simulink model "radia_ltspice_pid_optuna"  (R2026a)
settings: Solver=FixedStepDiscrete  StopTime=0.80000000000000004  FixedStep=0.1
settings Model: Creator=Administrator  LastModifiedBy=Administrator

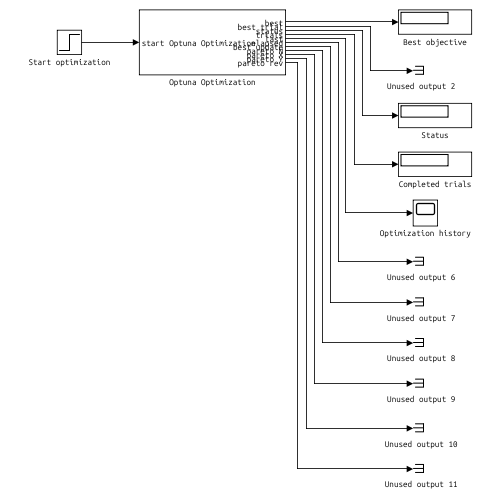
[thumbnail: Simulink's stored preview of the top-level diagram]
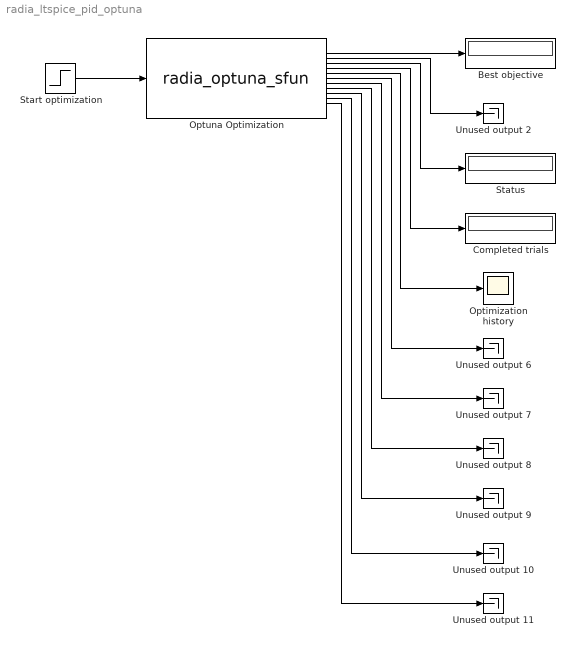
== system radia_ltspice_pid_optuna ==
  Best objective : Display
  Completed trials : Display
  Optimization history : Scope
  Optuna Optimization : M-S-Function  FunctionName=radia_optuna_sfun  Parameters=objective_fcn,num_trials,directions,storage_path,sample_time_s,strcmp(live_visualization,'on'),sampler_name  mask{objective_fcn='radia.simulink.ltspicePIDObjective', num_trials=8, directions="minimize", storage_path='', sample_time_s=0.10000000000000001, live_visualization=off, sampler_name=cmaes}
      mask prompts: objective_fcn "Objective function"; num_trials "Number of trials"; directions "Objective directions"; storage_path "Study MAT file"; sample_time_s "Trial sample time (s)"; live_visualization "External MATLAB monitor"; sampler_name "Sampler"
      mask help: Incremental MATLAB Optuna study. One trial executes per sample; connect the live outputs to an Optuna Monitor.
      mask TypeOptions sampler_name: auto | random | tpe | cmaes | motpe | nsgaii
      mask Display: disp('Optuna Optimization');port_label('input',1,'start');port_label('output',1,'best');port_label('output',2,'best trial');port_label('output',3,'status');port_label('output',4,'trials');port_label('output',5,'last');port_label('output',6,'elapsed');port_label('output',7,'best update');port_label('output',8,'pareto N');port_label('output',9,'pareto X');port_label('output',10,'pareto Y');port_label('output',11,'pareto rev');
  Start optimization : Step  Time=0  SampleTime=0.1
  Status : Display
  Unused output {2,6..11} (7 alike) : Terminator
  wires:
  Start optimization/1 -> Optuna Optimization/1
  Optuna Optimization/1 -> Best objective/1
  Optuna Optimization/2 -> Unused output 2/1
  Optuna Optimization/4 -> Completed trials/1
  Optuna Optimization/3 -> Status/1
  Optuna Optimization/10 -> Unused output 10/1
  Optuna Optimization/5 -> Optimization history/1
  Optuna Optimization/7 -> Unused output 7/1
  Optuna Optimization/6 -> Unused output 6/1
  Optuna Optimization/8 -> Unused output 8/1
  Optuna Optimization/9 -> Unused output 9/1
  Optuna Optimization/11 -> Unused output 11/1
